simulink model "rlQubeServo"  (R2018b)
settings: Solver=ode23t  StartTime=0.0  StopTime=10.0  RelTol=1e-3  AbsTol=1e-3
undefined symbols (not defined in the file): D_p, D_r_2, dphi0, dphi_gain, dtheta0, dtheta_gain, K_b_2, K_t, L_m, L_p, L_r, m_p, m_r, mu_m, n, p_rad, phi0, phi_gain, R_m, rod_rad, Tf, theta0, theta_gain, Ts, Volt_Limit, X, Y, Z
libraries: sm_lib x21, fl_lib x10, nesl_utility x9, rllib x2, simulink x2, ee_lib x1
(part 2 of 2)

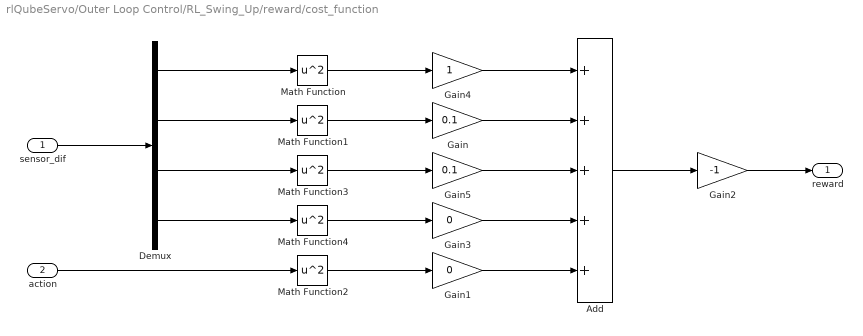
== system rlQubeServo/Outer Loop Control/RL_Swing_Up/reward/cost_function ==
  sensor_dif : Inport
  action : Inport  Port=2
  Add : Sum  Inputs=+++++
  Demux : Demux
  Gain : Gain  Gain=0.1
  Gain1 : Gain  Gain=0
  Gain2 : Gain  Gain=-1
  Gain3 : Gain  Gain=0
  Gain4 : Gain
  Gain5 : Gain  Gain=0.1
  Math Function{,1..4} (5 alike) : Math  Operator=square  SaturateOnIntegerOverflow=on
  reward : Outport
  wires:
  Math Function4/1 -> Gain3/1
  Gain4/1 -> Add/1
  Gain/1 -> Add/2
  Gain5/1 -> Add/3
  Gain3/1 -> Add/4
  Gain1/1 -> Add/5
  Gain2/1 -> reward/1
  Add/1 -> Gain2/1
  sensor_dif/1 -> Demux/1
  Demux/4 -> Math Function4/1
  Demux/3 -> Math Function3/1
  Demux/2 -> Math Function1/1
  Math Function1/1 -> Gain/1
  Math Function3/1 -> Gain5/1
  action/1 -> Math Function2/1
  Demux/1 -> Math Function/1
  Math Function/1 -> Gain4/1
  Math Function2/1 -> Gain1/1

== system rlQubeServo/Outer Loop Control/RL_Swing_Up/reward/failure_cost ==
  isdone_flag : Inport
  Add : Sum
  Constant1 : Constant  Value=0
  Constant2 : Constant  Value=0
  Constant7 : Constant  Value=0
  Gain1 : Gain  Gain=-1
  Gain2 : Gain  Gain=Ts/Tf
  Switch : Switch  Criteria=u2 > Threshold
  reward : Outport
  wires:
  Gain1/1 -> Add/1
  Constant2/1 -> Switch/3
  Constant1/1 -> Switch/1
  isdone_flag/1 -> Switch/2
  Switch/1 -> Gain1/1
  Gain2/1 -> Add/2
  Add/1 -> reward/1
  Constant7/1 -> Gain2/1

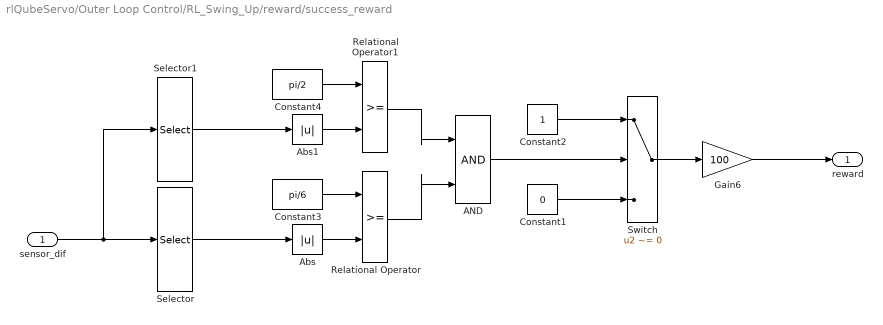
== system rlQubeServo/Outer Loop Control/RL_Swing_Up/reward/success_reward ==
  sensor_dif : Inport
  AND : Logic  IconShape=distinctive  AllPortsSameDT=off  OutDataTypeStr=boolean
  Abs : Abs
  Abs1 : Abs
  Constant1 : Constant  Value=0
  Constant2 : Constant
  Constant3 : Constant  Value=pi/6
  Constant4 : Constant  Value=pi/2
  Gain6 : Gain  Gain=100
  Relational Operator : RelationalOperator  OutDataTypeStr=boolean  RndMeth=Simplest
  Relational Operator1 : RelationalOperator  OutDataTypeStr=boolean  RndMeth=Simplest
  Selector : Selector  InputPortWidth=4  IndexOptions=Index vector (dialog)  Indices=[2]  OutputSizes=1
  Selector1 : Selector  InputPortWidth=4  IndexOptions=Index vector (dialog)  Indices=[1]  OutputSizes=1
  Switch : Switch  Criteria=u2 ~= 0
  reward : Outport
  wires:
  sensor_dif/1 -> Selector1/1, Selector/1
  Gain6/1 -> reward/1
  Selector/1 -> Abs/1
  Constant2/1 -> Switch/1
  Constant1/1 -> Switch/3
  Switch/1 -> Gain6/1
  Constant3/1 -> Relational Operator/1
  Abs/1 -> Relational Operator/2
  AND/1 -> Switch/2
  Relational Operator/1 -> AND/2
  Abs1/1 -> Relational Operator1/2
  Constant4/1 -> Relational Operator1/1
  Relational Operator1/1 -> AND/1
  Selector1/1 -> Abs1/1

== system rlQubeServo/Qube servo/Pendulum Physical Model/stopper/stopper_off ==
  Conn1 : PMIOPort  Side=Left
  Conn2 : PMIOPort  Port=2  Side=Right

== system rlQubeServo/Qube servo/Pendulum Physical Model/stopper/stopper_on ==
  Spatial Contact Force : sm_lib/Forces and Torques/Spatial Contact Force  NormalForceType=SmoothSpringDamper  NormalStiffness=1e6  NormalStiffnessUnits=N/m  NormalDamping=1e3  NormalDampingUnits=N/(m/s)  NormalTransitionRegionWidth=1e-4  NormalTransitionRegionWidthUnits=m  FrictionType=SmoothStickSlip  CoefficientOfStaticFriction=0.5  CoefficientOfDynamicFriction=0.3  FrictionalCriticalVelocity=1e-3  FrictionalCriticalVelocityUnits=m/s  SenseContactSignal=off  SensePenetrationDepth=off  SenseSeparationDistance=off  SenseNormalForceMagnitude=off  SenseFrictionalForceMagnitude=off  SenseNormalVelocity=off  SenseTangentialVelocity=off  SenseContactBaseRotation=off  SenseContactBaseTranslation=off  SenseContactFollowerRotation=off  SenseContactFollowerTranslation=off  ZeroCrossDetectContactStartAndEnd=off
  Conn1 : PMIOPort  Side=Left
  Conn2 : PMIOPort  Port=2  Side=Right
  connections:
  Spatial Contact Force/RConn1 -- Conn2/RConn1
  Conn1/RConn1 -- Spatial Contact Force/LConn1

== system rlQubeServo/Outer Loop Control/RL_Mode_Select/reward/change_angle_range/change_angle_range ==
  In_angle : Inport
  Constant3 : Constant  Value=pi  OutDataTypeStr=Inherit: Inherit via back propagation
  Constant4 : Constant  Value=2*pi  OutDataTypeStr=Inherit: Inherit via back propagation
  Constant6 : Constant  Value=-pi  OutDataTypeStr=Inherit: Inherit via back propagation
  Relational Operator2 : RelationalOperator  Operator=<  OutDataTypeStr=boolean  RndMeth=Nearest
  Relational Operator3 : RelationalOperator  Operator=>  OutDataTypeStr=boolean  RndMeth=Nearest
  Sum10 : Sum  Inputs=|++
  Sum9 : Sum  Inputs=|+-
  Switch8 : Switch  Criteria=u2 ~= 0
  Switch9 : Switch  Criteria=u2 ~= 0
  Out_angle : Outport
  wires:
  Switch9/1 -> Out_angle/1
  Sum9/1 -> Switch8/3
  Switch8/1 -> Switch9/1, Sum10/1, Relational Operator3/1
  Sum10/1 -> Switch9/3
  Constant4/1 -> Sum9/2, Sum10/2
  Constant3/1 -> Relational Operator2/2
  Relational Operator3/1 -> Switch9/2
  In_angle/1 -> Switch8/1, Sum9/1, Relational Operator2/1
  Relational Operator2/1 -> Switch8/2
  Constant6/1 -> Relational Operator3/2

== system rlQubeServo/Outer Loop Control/RL_Mode_Select/reward/change_angle_range/change_angle_range1 ==
  In_angle : Inport
  Constant3 : Constant  Value=pi  OutDataTypeStr=Inherit: Inherit via back propagation
  Constant4 : Constant  Value=2*pi  OutDataTypeStr=Inherit: Inherit via back propagation
  Constant6 : Constant  Value=-pi  OutDataTypeStr=Inherit: Inherit via back propagation
  Relational Operator2 : RelationalOperator  Operator=<  OutDataTypeStr=boolean  RndMeth=Nearest
  Relational Operator3 : RelationalOperator  Operator=>  OutDataTypeStr=boolean  RndMeth=Nearest
  Sum10 : Sum  Inputs=|++
  Sum9 : Sum  Inputs=|+-
  Switch8 : Switch  Criteria=u2 ~= 0
  Switch9 : Switch  Criteria=u2 ~= 0
  Out_angle : Outport
  wires:
  Switch9/1 -> Out_angle/1
  Sum9/1 -> Switch8/3
  Switch8/1 -> Switch9/1, Sum10/1, Relational Operator3/1
  Sum10/1 -> Switch9/3
  Constant4/1 -> Sum9/2, Sum10/2
  Constant3/1 -> Relational Operator2/2
  Relational Operator3/1 -> Switch9/2
  In_angle/1 -> Switch8/1, Sum9/1, Relational Operator2/1
  Relational Operator2/1 -> Switch8/2
  Constant6/1 -> Relational Operator3/2

== system rlQubeServo/Outer Loop Control/RL_Mode_Select/reward/change_angle_range/mod_2pi ==
  In_angle : Inport
  MATLAB Function : MATLAB Function  TreatAsAtomicUnit=on
  Out_angle : Outport
  wires:
  In_angle/1 -> MATLAB Function/1(u)
  MATLAB Function/1(y) -> Out_angle/1

== system rlQubeServo/Outer Loop Control/RL_Mode_Select/reward/change_angle_range/mod_2pi1 ==
  In_angle : Inport
  MATLAB Function : MATLAB Function  TreatAsAtomicUnit=on
  Out_angle : Outport
  wires:
  In_angle/1 -> MATLAB Function/1(u)
  MATLAB Function/1(y) -> Out_angle/1

== system rlQubeServo/Outer Loop Control/RL_Swing_Up/reward/change_angle_range/change_angle_range ==
  In_angle : Inport
  Constant3 : Constant  Value=pi  OutDataTypeStr=Inherit: Inherit via back propagation
  Constant4 : Constant  Value=2*pi  OutDataTypeStr=Inherit: Inherit via back propagation
  Constant6 : Constant  Value=-pi  OutDataTypeStr=Inherit: Inherit via back propagation
  Relational Operator2 : RelationalOperator  Operator=<  OutDataTypeStr=boolean  RndMeth=Nearest
  Relational Operator3 : RelationalOperator  Operator=>  OutDataTypeStr=boolean  RndMeth=Nearest
  Sum10 : Sum  Inputs=|++
  Sum9 : Sum  Inputs=|+-
  Switch8 : Switch  Criteria=u2 ~= 0
  Switch9 : Switch  Criteria=u2 ~= 0
  Out_angle : Outport
  wires:
  Switch9/1 -> Out_angle/1
  Sum9/1 -> Switch8/3
  Switch8/1 -> Switch9/1, Sum10/1, Relational Operator3/1
  Sum10/1 -> Switch9/3
  Constant4/1 -> Sum9/2, Sum10/2
  Constant3/1 -> Relational Operator2/2
  Relational Operator3/1 -> Switch9/2
  In_angle/1 -> Switch8/1, Sum9/1, Relational Operator2/1
  Relational Operator2/1 -> Switch8/2
  Constant6/1 -> Relational Operator3/2

== system rlQubeServo/Outer Loop Control/RL_Swing_Up/reward/change_angle_range/change_angle_range1 ==
  In_angle : Inport
  Constant3 : Constant  Value=pi  OutDataTypeStr=Inherit: Inherit via back propagation
  Constant4 : Constant  Value=2*pi  OutDataTypeStr=Inherit: Inherit via back propagation
  Constant6 : Constant  Value=-pi  OutDataTypeStr=Inherit: Inherit via back propagation
  Relational Operator2 : RelationalOperator  Operator=<  OutDataTypeStr=boolean  RndMeth=Nearest
  Relational Operator3 : RelationalOperator  Operator=>  OutDataTypeStr=boolean  RndMeth=Nearest
  Sum10 : Sum  Inputs=|++
  Sum9 : Sum  Inputs=|+-
  Switch8 : Switch  Criteria=u2 ~= 0
  Switch9 : Switch  Criteria=u2 ~= 0
  Out_angle : Outport
  wires:
  Switch9/1 -> Out_angle/1
  Sum9/1 -> Switch8/3
  Switch8/1 -> Switch9/1, Sum10/1, Relational Operator3/1
  Sum10/1 -> Switch9/3
  Constant4/1 -> Sum9/2, Sum10/2
  Constant3/1 -> Relational Operator2/2
  Relational Operator3/1 -> Switch9/2
  In_angle/1 -> Switch8/1, Sum9/1, Relational Operator2/1
  Relational Operator2/1 -> Switch8/2
  Constant6/1 -> Relational Operator3/2

== system rlQubeServo/Outer Loop Control/RL_Swing_Up/reward/change_angle_range/mod_2pi ==
  In_angle : Inport
  MATLAB Function : MATLAB Function  TreatAsAtomicUnit=on
  Out_angle : Outport
  wires:
  In_angle/1 -> MATLAB Function/1(u)
  MATLAB Function/1(y) -> Out_angle/1

== system rlQubeServo/Outer Loop Control/RL_Swing_Up/reward/change_angle_range/mod_2pi1 ==
  In_angle : Inport
  MATLAB Function : MATLAB Function  TreatAsAtomicUnit=on
  Out_angle : Outport
  wires:
  In_angle/1 -> MATLAB Function/1(u)
  MATLAB Function/1(y) -> Out_angle/1

== matlab function rlQubeServo/Inner Loop Control/mod_2pi/MATLAB Function ==
  data: u input; y output
function y = fcn(u)

TWO_PI = 2*pi;
input = u;

if (input >= 0)
    while (input > TWO_PI)
        input = input - TWO_PI;
    end
else
    while (input < -TWO_PI)
        input = input + TWO_PI;
    end
end

y = input;

end

== matlab function rlQubeServo/Inner Loop Control/change_angle1/mod_2pi/MATLAB Function ==
  data: u input; y output
function y = fcn(u)

TWO_PI = 2*pi;
input = u;

if (input >= 0)
    while (input > TWO_PI)
        input = input - TWO_PI;
    end
else
    while (input < -TWO_PI)
        input = input + TWO_PI;
    end
end

y = input;

end

== matlab function rlQubeServo/Inner Loop Control/change_angle/mod_2pi/MATLAB Function ==
  data: u input; y output
function y = fcn(u)

TWO_PI = 2*pi;
input = u;

if (input >= 0)
    while (input > TWO_PI)
        input = input - TWO_PI;
    end
else
    while (input < -TWO_PI)
        input = input + TWO_PI;
    end
end

y = input;

end

== matlab function rlQubeServo/Outer Loop Control/RL_Swing_Up/reward/change_angle_range/mod_2pi/MATLAB Function ==
  data: u input; y output
function y = fcn(u)

TWO_PI = 2*pi;
input = u;

if (input >= 0)
    while (input > TWO_PI)
        input = input - TWO_PI;
    end
else
    while (input < -TWO_PI)
        input = input + TWO_PI;
    end
end

y = input;

end

== matlab function rlQubeServo/Outer Loop Control/RL_Swing_Up/reward/change_angle_range/mod_2pi1/MATLAB Function ==
  data: u input; y output
function y = fcn(u)

TWO_PI = 2*pi;
input = u;

if (input >= 0)
    while (input > TWO_PI)
        input = input - TWO_PI;
    end
else
    while (input < -TWO_PI)
        input = input + TWO_PI;
    end
end

y = input;

end

== matlab function rlQubeServo/Outer Loop Control/RL_Mode_Select/reward/change_angle_range/mod_2pi/MATLAB Function ==
  data: u input; y output
function y = fcn(u)

TWO_PI = 2*pi;
input = u;

if (input >= 0)
    while (input > TWO_PI)
        input = input - TWO_PI;
    end
else
    while (input < -TWO_PI)
        input = input + TWO_PI;
    end
end

y = input;

end

== matlab function rlQubeServo/Outer Loop Control/RL_Mode_Select/reward/change_angle_range/mod_2pi1/MATLAB Function ==
  data: u input; y output
function y = fcn(u)

TWO_PI = 2*pi;
input = u;

if (input >= 0)
    while (input > TWO_PI)
        input = input - TWO_PI;
    end
else
    while (input < -TWO_PI)
        input = input + TWO_PI;
    end
end

y = input;

end
